simulink model "forward_kinematics_func_sim"  (R2023a)
settings: Solver=VariableStepAuto  StartTime=0.0  StopTime=10.0  RelTol=1e-3
settings Model: Creator=totae  LastModifiedBy=totae

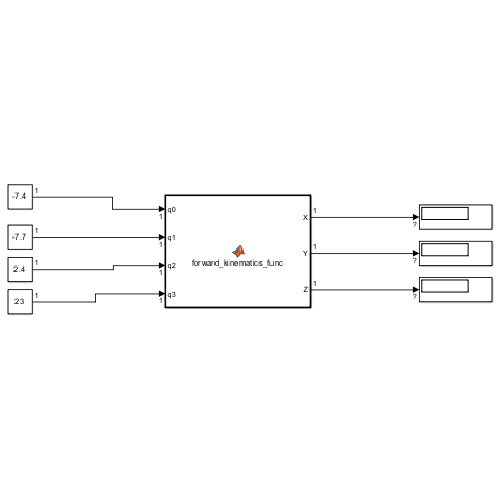
[thumbnail: Simulink's stored preview of the top-level diagram]
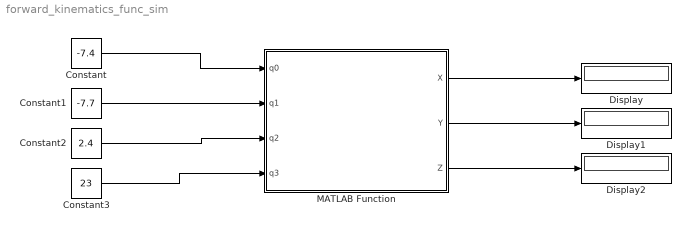
== system forward_kinematics_func_sim ==
  Constant : Constant  Value=-7.4
  Constant1 : Constant  Value=-7.7
  Constant2 : Constant  Value=2.4
  Constant3 : Constant  Value=23
  Display : Display
  Display1 : Display
  Display2 : Display
  MATLAB Function : MATLAB Function  TreatAsAtomicUnit=on
  wires:
  MATLAB Function/1(X) -> Display/1
  MATLAB Function/2(Y) -> Display1/1
  MATLAB Function/3(Z) -> Display2/1
  Constant/1 -> MATLAB Function/1(q0)
  Constant1/1 -> MATLAB Function/2(q1)
  Constant2/1 -> MATLAB Function/3(q2)
  Constant3/1 -> MATLAB Function/4(q3)

== matlab function forward_kinematics_func_sim/MATLAB Function ==
  data: q0 input; X output; q1 input; q2 input; q3 input; Y output; Z output
function [X,Y,Z] = forward_kinematics_func(q0,q1,q2,q3)
%UNTITLED Summary of this function goes here
%  obtain the position of the end effector from...
% the multiplication of the transformation functions

T1=transformation_func(q0,0.066,0,(pi/2));
T2=transformation_func((-(pi/2)+q1),0,0,(pi/2));
T3=transformation_func((-(pi/2)+q2),0.149,0,(pi/2));
T4=transformation_func((-(pi/2)+q3),0,0.144,0);

T_EE=T1*T2*T3*T4;
X=T_EE(1,4);
Y=T_EE(2,4);
Z=T_EE(3,4);

% X=vpa(X,3);
% Y=vpa(Y,3);
% Z=vpa(Z,3);
% T10=transformation_func(0,-0.066,0,(-pi/2));
% T20=transformation_func(((-pi/2)+0),0,0,(pi/2));
% T30=transformation_func(((-pi/2)+0),-0.149,0,(pi/2));
% T40=transformation_func(((-pi/2)+0),0,0.152,0);
% 
% T_EE0=T10*T20*T30*T40;
% X0=T_EE0(1,4)
% Y0=T_EE0(2,4)
% Z0=T_EE0(3,4)

% if abs(X) < 1e-10
%     X=0;
% elseif abs(Y)< 1e-10
%      Y=0;
%  elseif abs(Z)< 1e-10
%      Z=0;    
% end
% xvec=[X0,X];
% yvec=[Y0,Y];
% zvec=[Z0,Z];

%plot3(X,Y,Z,'r*')
end
